simulink library "SUB_L4_Task_10ms_SUB_VELOCITYDISTCTRL"  (R2018a)
settings: Solver=VariableStepAuto  StartTime=0.0  StopTime=10.0  RelTol=1e-3
undefined symbols (not defined in the file or in its folder): DiscIntNeverNeededParam, ENUM_XBR_CONTROL_MODE_T, ENUM_XBR_EBI_MODE_T, ENUM_XBR_PASS_THROUGH_ACTIVE_T, ENUM_XBR_PRIORITY_T, magnitude
libraries: EmE_MBD_Blockset x14, simulink x6, PTC_MBDS_LIB x1
settings Model: Creator=Chris.Balton  LastModifiedBy=Chris.Balton

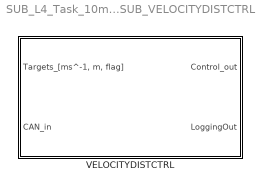
== system SUB_L4_Task_10ms_SUB_VELOCITYDISTCTRL ==
  VELOCITYDISTCTRL : Subsystem

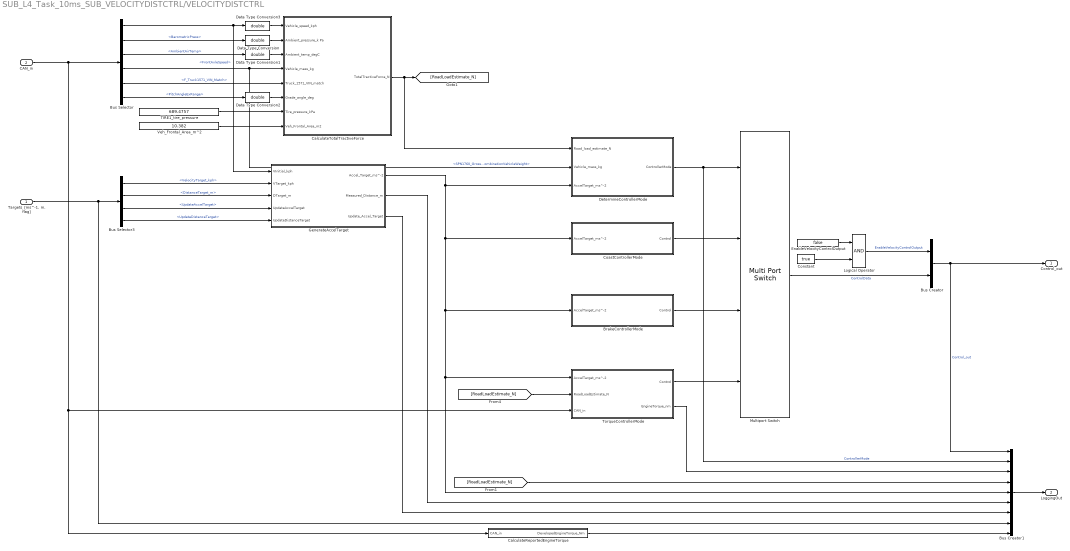
== system SUB_L4_Task_10ms_SUB_VELOCITYDISTCTRL/VELOCITYDISTCTRL ==
  "Targets_[ms^-1, m, flag]" : Inport
  CAN_in : Inport  Port=2
  BrakeControllerMode : Subsystem
  Bus Creator : BusCreator  Inputs=2
  Bus Creator1 : BusCreator  Inputs=9
  Bus Selector : BusSelector  OutputSignals=CAN.EBC2_0B.FrontAxleSpeed,CAN.AMB_00.BarometricPress,CAN.AMB_00.AmbientAirTemp,CAN.CVW_0B.SPN1760_GrossCombinationVehicleWeight,CAN.VI_00.F_Truck1571_VIN_Match,CAN.SSI2_03.PitchAngleExRange
  Bus Selector3 : BusSelector  OutputSignals=VelocityTarget_kph,DistanceTarget_m,UpdateAccelTarget,UpdateDistanceTarget
  CalculateReportedEngineTorque : Subsystem
  CalculateTotalTractiveForce : Subsystem
  CoastControllerMode : Subsystem
  Constant : Constant  Value=true  OutDataTypeStr=boolean
  Data Type Conversion{,1..3} (4 alike) : DataTypeConversion  OutDataTypeStr=double
      settings: AttributesFormatString=%<OutDataTypeStr>
  DetermineControllerMode : Subsystem
  EnableVelocityControlOutput : Constant  Value=false  OutDataTypeStr=boolean
  GenerateAccelTarget : Subsystem
  Logical Operator : Logic  OutDataTypeStr=boolean
  Multiport Switch : MultiPortSwitch
  TIRE1_tire_pressure : Constant  Value=689.4757
  TorqueControllerMode : Subsystem
  Veh_Frontal_Area_m^2 : Constant  Value=10.382
  Control_out : Outport
  LoggingOut : Outport  Port=2
  wires:
  Bus Selector3/4 -> GenerateAccelTarget/5(UpdateDistanceTarget)  "<UpdateDistanceTarget>"
  [RoadLoadEstimate_N] -> Bus Creator1/4
  CalculateReportedEngineTorque/1(DevelopedEngineTorque_Nm) -> Bus Creator1/9
  GenerateAccelTarget/2(Measured_Distance_m) -> Bus Creator1/6
  GenerateAccelTarget/3(Update_Accel_Target) -> Bus Creator1/7
  Constant/1 -> Logical Operator/2
  EnableVelocityControlOutput/1 -> Logical Operator/1
  Bus Creator1/1 -> LoggingOut/1
  TorqueControllerMode/2(EngineTorque_nm) -> Bus Creator1/3
  Logical Operator/1 -> Bus Creator/1  "EnableVelocityControlOutput"
  Bus Creator/1 -> Control_out/1, Bus Creator1/1  "Control_out"
  CAN_in/1 -> Bus Selector/1, CalculateReportedEngineTorque/1(CAN_in), TorqueControllerMode/3(CAN_in)
  Bus Selector/4 -> DetermineControllerMode/2(Vehicle_mass_kg), CalculateTotalTractiveForce/4(Vehicle_mass_kg)  "<SPN1760_GrossCombinationVehicleWeight>"
  Bus Selector/3 -> Data Type Conversion1/1  "<AmbientAirTemp>"
  Bus Selector3/3 -> GenerateAccelTarget/4(UpdateAccelTarget)  "<UpdateAccelTarget>"
  Data Type Conversion3/1 -> CalculateTotalTractiveForce/1(Vehicle_speed_kph)
  Bus Selector/1 -> Data Type Conversion3/1, GenerateAccelTarget/1(VInitial_kph)  "<FrontAxleSpeed>"
  Data Type Conversion1/1 -> CalculateTotalTractiveForce/3(Ambient_temp_degC)
  Data Type Conversion/1 -> CalculateTotalTractiveForce/2(Ambient_pressure_k Pa)
  Bus Selector3/2 -> GenerateAccelTarget/3(DTarget_m)  "<DistanceTarget_m>"
  Bus Selector3/1 -> GenerateAccelTarget/2(VTarget_kph)  "<VelocityTarget_kph>"
  Bus Selector/6 -> Data Type Conversion2/1  "<PitchAngleExRange>"
  TIRE1_tire_pressure/1 -> CalculateTotalTractiveForce/7(Tire_pressure_kPa)
  Veh_Frontal_Area_m^2/1 -> CalculateTotalTractiveForce/8(Veh_Frontal_Area_m2)
  "Targets_[ms^-1, m, flag]"/1 -> Bus Creator1/8, Bus Selector3/1
  Bus Selector/5 -> CalculateTotalTractiveForce/5(Truck_1571_VIN_match)  "<F_Truck1571_VIN_Match>"
  Bus Selector/2 -> Data Type Conversion/1  "<BarometricPress>"
  DetermineControllerMode/1(ControllerMode) -> Multiport Switch/1, Bus Creator1/2  "ControllerMode"
  GenerateAccelTarget/1(Accel_Target_ms^-2) -> Bus Creator1/5, TorqueControllerMode/1(AccelTarget_ms^-2), BrakeControllerMode/1(AccelTarget_ms^-2), CoastControllerMode/1(AccelTarget_ms^-2), DetermineControllerMode/3(AccelTarget_ms^-2)
  [RoadLoadEstimate_N] -> TorqueControllerMode/2(RoadLoadEstimate_N)
  CalculateTotalTractiveForce/1(TotalTractiveForce_N) -> DetermineControllerMode/1(Road_load_estimate_N), [RoadLoadEstimate_N]
  Multiport Switch/1 -> Bus Creator/2  "ControlData"
  TorqueControllerMode/1(Control) -> Multiport Switch/4
  BrakeControllerMode/1(Control) -> Multiport Switch/3
  CoastControllerMode/1(Control) -> Multiport Switch/2
  Data Type Conversion2/1 -> CalculateTotalTractiveForce/6(Grade_angle_deg)

== system SUB_L4_Task_10ms_SUB_VELOCITYDISTCTRL/VELOCITYDISTCTRL/BrakeControllerMode ==
  AccelTarget_ms^-2 : Inport
  Accel_pedal_coast : Constant  Value=0
  Bus Creator : BusCreator  Inputs=2
  Bus Creator1 : BusCreator  Inputs=7
  Gain : Gain
  XBRControlMode : Constant  Value=ENUM_XBR_CONTROL_MODE_T.ACCEL_CTRL_WITH_MAX_MODE
  XBREnduranceBrakeIntegrationMode : Constant  Value=ENUM_XBR_EBI_MODE_T.EBI_ALLOWED
  XBRPassThroughActiveOVR : Constant  Value=ENUM_XBR_PASS_THROUGH_ACTIVE_T.ACTIVE
  XBRPassThroughEnabled : Constant
  XBRPriority : Constant  Value=ENUM_XBR_PRIORITY_T.MEDIUM_PRIORITY
  XBRUrgency : Constant  Value=25
  Control : Outport
  wires:
  AccelTarget_ms^-2/1 -> Gain/1  "AccelTarget_ms^-2"
  Bus Creator1/1 -> Bus Creator/1  "XBR_data"
  Gain/1 -> Bus Creator1/1  "XBRExternalAccelDemand"
  XBRPassThroughActiveOVR/1 -> Bus Creator1/5  "XBRPassThroughActive"
  XBREnduranceBrakeIntegrationMode/1 -> Bus Creator1/2  "XBREnduranceBrakeIntegrationMode"
  XBRUrgency/1 -> Bus Creator1/6  "XBRUrgency"
  XBRControlMode/1 -> Bus Creator1/4  "XBRControlMode"
  XBRPriority/1 -> Bus Creator1/3  "XBRPriority"
  XBRPassThroughEnabled/1 -> Bus Creator1/7  "XBRPassThroughEnabled"
  Bus Creator/1 -> Control/1  "ControlData"
  Accel_pedal_coast/1 -> Bus Creator/2  "AcceleratorPedalPosOut"

== system SUB_L4_Task_10ms_SUB_VELOCITYDISTCTRL/VELOCITYDISTCTRL/CalculateReportedEngineTorque ==
  CAN_in : Inport
  Add : Sum  OutDataTypeStr=double  InputSameDT=on
  Bus Selector : BusSelector  OutputSignals=CAN.EC1_00.SPN544_EngineReferenceTorque,CAN.EEC1_00.ActlEngPrcntTrqueHighResolution,CAN.EEC1_00.ActualEngPercentTorque
  ConvToPercent : Constant  Value=0.01
  Data Type Conversion : DataTypeConversion  OutDataTypeStr=double
  Product : Product  Inputs=3  InputSameDT=on
  DevelopedEngineTorque_Nm : Outport
      settings: AttributesFormatString=IC: %<InitialOutput>\nDisabled value: %<OutputWhenDisabled>
  wires:
  ConvToPercent/1 -> Product/3
  Product/1 -> DevelopedEngineTorque_Nm/1  "DevelopedEngineTorque_Nm"
  Add/1 -> Product/2  "EnginePercentTorque"
  Bus Selector/3 -> Add/2  "<ActualEngPercentTorque>"
  Bus Selector/2 -> Add/1  "<ActlEngPrcntTrqueHighResolution>"
  Bus Selector/1 -> Data Type Conversion/1  "<SPN544_EngineReferenceTorque>"
  CAN_in/1 -> Bus Selector/1
  Data Type Conversion/1 -> Product/1

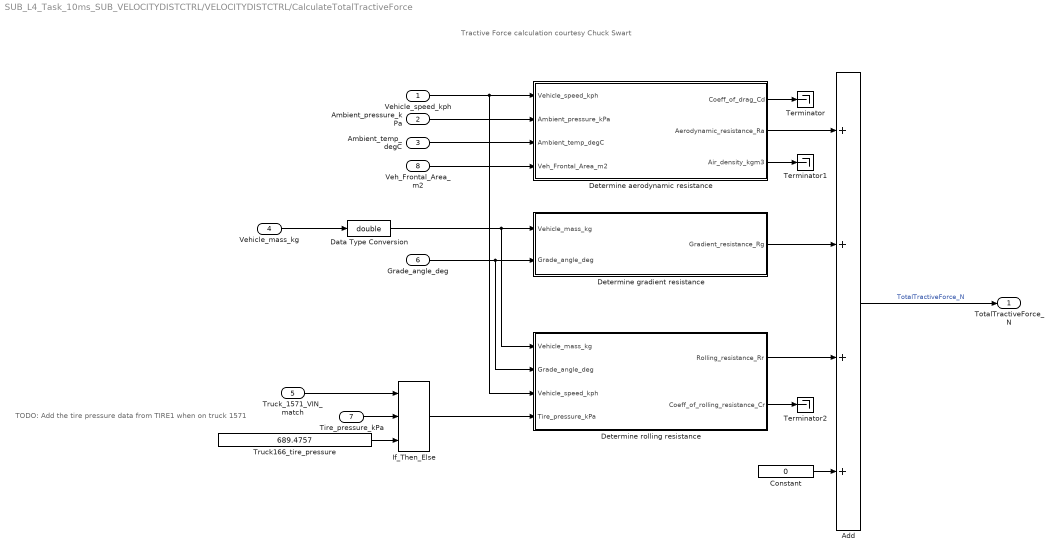
== system SUB_L4_Task_10ms_SUB_VELOCITYDISTCTRL/VELOCITYDISTCTRL/CalculateTotalTractiveForce ==
  note: TODO: Add the tire pressure data from TIRE1 when on truck 1571
  note: Tractive Force calculation courtesy Chuck Swart
  Vehicle_speed_kph : Inport
  Ambient_pressure_k Pa : Inport  Port=2
  Ambient_temp_degC : Inport  Port=3
  Vehicle_mass_kg : Inport  Port=4
  Truck_1571_VIN_match : Inport  Port=5
  Grade_angle_deg : Inport  Port=6
  Tire_pressure_kPa : Inport  Port=7
  Veh_Frontal_Area_m2 : Inport  Port=8
  Add : Sum  Inputs=++++  InputSameDT=on
  Constant : Constant  Value=0
  Data Type Conversion : DataTypeConversion  OutDataTypeStr=double
  Determine aerodynamic resistance : Subsystem
  Determine gradient resistance : Subsystem
  Determine rolling resistance : Subsystem
  If_Then_Else : EmE_MBD_Blockset/Signal Routing/If_Then_Else
      settings: SourceProductName=PACCAR EmE MBD Blockset
  Terminator : Terminator
  Terminator1 : Terminator
  Terminator2 : Terminator
  Truck166_tire_pressure : Constant  Value=689.4757
  TotalTractiveForce_N : Outport
  wires:
  If_Then_Else/1 -> Determine rolling resistance/4(Tire_pressure_kPa)
  Determine rolling resistance/2(Coeff_of_rolling_resistance_Cr) -> Terminator2/1
  Determine rolling resistance/1(Rolling_resistance_Rr) -> Add/3
  Ambient_pressure_k Pa/1 -> Determine aerodynamic resistance/2(Ambient_pressure_kPa)
  Add/1 -> TotalTractiveForce_N/1  "TotalTractiveForce_N"
  Vehicle_speed_kph/1 -> Determine rolling resistance/3(Vehicle_speed_kph), Determine aerodynamic resistance/1(Vehicle_speed_kph)
  Ambient_temp_degC/1 -> Determine aerodynamic resistance/3(Ambient_temp_degC)
  Determine aerodynamic resistance/1(Coeff_of_drag_Cd) -> Terminator/1
  Veh_Frontal_Area_m2/1 -> Determine aerodynamic resistance/4(Veh_Frontal_Area_m2)
  Constant/1 -> Add/4
  Vehicle_mass_kg/1 -> Data Type Conversion/1
  Grade_angle_deg/1 -> Determine rolling resistance/2(Grade_angle_deg), Determine gradient resistance/2(Grade_angle_deg)
  Determine gradient resistance/1(Gradient_resistance_Rg) -> Add/2
  Determine aerodynamic resistance/3(Air_density_kgm3) -> Terminator1/1
  Determine aerodynamic resistance/2(Aerodynamic_resistance_Ra) -> Add/1
  Tire_pressure_kPa/1 -> If_Then_Else/2
  Truck166_tire_pressure/1 -> If_Then_Else/3
  Truck_1571_VIN_match/1 -> If_Then_Else/1
  Data Type Conversion/1 -> Determine rolling resistance/1(Vehicle_mass_kg), Determine gradient resistance/1(Vehicle_mass_kg)

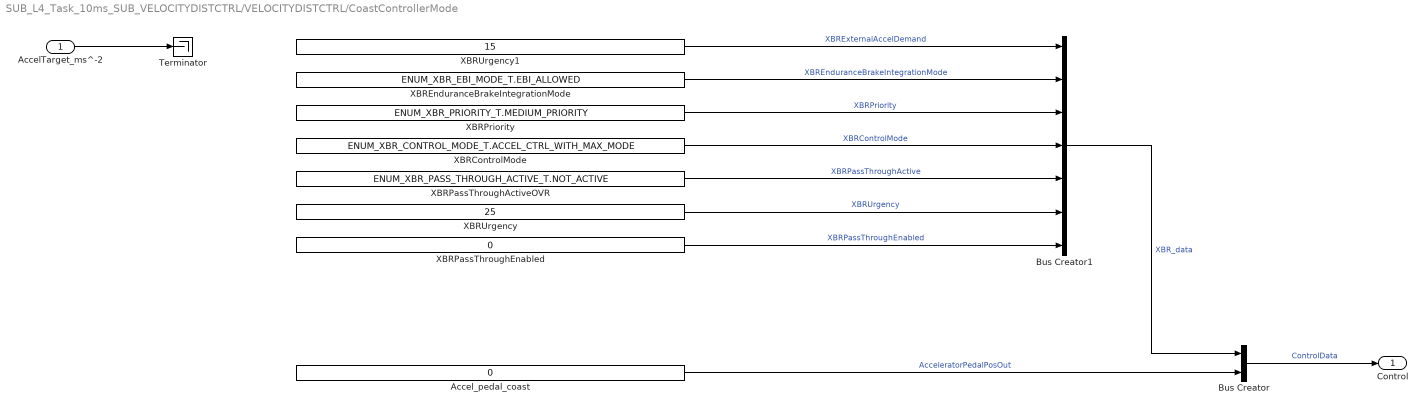
== system SUB_L4_Task_10ms_SUB_VELOCITYDISTCTRL/VELOCITYDISTCTRL/CoastControllerMode ==
  AccelTarget_ms^-2 : Inport
  Accel_pedal_coast : Constant  Value=0
  Bus Creator : BusCreator  Inputs=2
  Bus Creator1 : BusCreator  Inputs=7
  Terminator : Terminator
  XBRControlMode : Constant  Value=ENUM_XBR_CONTROL_MODE_T.ACCEL_CTRL_WITH_MAX_MODE
  XBREnduranceBrakeIntegrationMode : Constant  Value=ENUM_XBR_EBI_MODE_T.EBI_ALLOWED
  XBRPassThroughActiveOVR : Constant  Value=ENUM_XBR_PASS_THROUGH_ACTIVE_T.NOT_ACTIVE
  XBRPassThroughEnabled : Constant  Value=0
  XBRPriority : Constant  Value=ENUM_XBR_PRIORITY_T.MEDIUM_PRIORITY
  XBRUrgency : Constant  Value=25
  XBRUrgency1 : Constant  Value=15
  Control : Outport
  wires:
  Bus Creator1/1 -> Bus Creator/1  "XBR_data"
  XBRUrgency1/1 -> Bus Creator1/1  "XBRExternalAccelDemand"
  XBRPassThroughActiveOVR/1 -> Bus Creator1/5  "XBRPassThroughActive"
  XBREnduranceBrakeIntegrationMode/1 -> Bus Creator1/2  "XBREnduranceBrakeIntegrationMode"
  XBRUrgency/1 -> Bus Creator1/6  "XBRUrgency"
  XBRControlMode/1 -> Bus Creator1/4  "XBRControlMode"
  XBRPriority/1 -> Bus Creator1/3  "XBRPriority"
  XBRPassThroughEnabled/1 -> Bus Creator1/7  "XBRPassThroughEnabled"
  AccelTarget_ms^-2/1 -> Terminator/1
  Bus Creator/1 -> Control/1  "ControlData"
  Accel_pedal_coast/1 -> Bus Creator/2  "AcceleratorPedalPosOut"

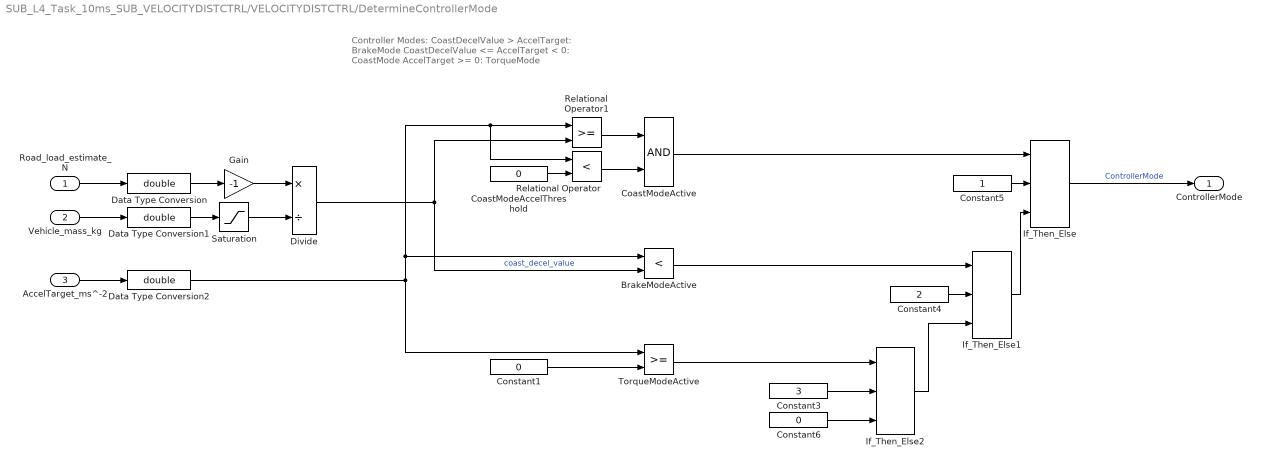
== system SUB_L4_Task_10ms_SUB_VELOCITYDISTCTRL/VELOCITYDISTCTRL/DetermineControllerMode ==
  note: Controller Modes:
      |
      | CoastDecelValue  >  AccelTarget:         BrakeMode
      | CoastDecelValue <= AccelTarget < 0:   CoastMode
      |                                  AccelTarget >= 0: TorqueMode
  Road_load_estimate_N : Inport
  Vehicle_mass_kg : Inport  Port=2
  AccelTarget_ms^-2 : Inport  Port=3
  BrakeModeActive : RelationalOperator  Operator=<  OutDataTypeStr=boolean  RndMeth=Nearest
  CoastModeAccelThreshold : Constant  Value=0
  CoastModeActive : Logic  AllPortsSameDT=off  OutDataTypeStr=boolean
  Constant1 : Constant  Value=0  SampleTime=-1
  Constant3 : Constant  Value=3  SampleTime=0.01
  Constant4 : Constant  Value=2  SampleTime=0.01
  Constant5 : Constant  SampleTime=0.01
  Constant6 : Constant  Value=0  SampleTime=0.01
  Data Type Conversion : DataTypeConversion  OutDataTypeStr=double
  Data Type Conversion1 : DataTypeConversion  OutDataTypeStr=double
  Data Type Conversion2 : DataTypeConversion  OutDataTypeStr=double
  Divide : Product  Inputs=*/  InputSameDT=on
  Gain : Gain  Gain=-1
  If_Then_Else : EmE_MBD_Blockset/Signal Routing/If_Then_Else
      settings: SourceProductName=PACCAR EmE MBD Blockset
  If_Then_Else1 : EmE_MBD_Blockset/Signal Routing/If_Then_Else
      settings: SourceProductName=PACCAR EmE MBD Blockset
  If_Then_Else2 : EmE_MBD_Blockset/Signal Routing/If_Then_Else
      settings: SourceProductName=PACCAR EmE MBD Blockset
  Relational Operator : RelationalOperator  Operator=<  OutDataTypeStr=boolean  RndMeth=Nearest
  Relational Operator1 : RelationalOperator  OutDataTypeStr=boolean  RndMeth=Nearest
  Saturation : Saturate  UpperLimit=50000  LowerLimit=1
  TorqueModeActive : RelationalOperator  OutDataTypeStr=boolean  RndMeth=Nearest
  ControllerMode : Outport
  wires:
  Road_load_estimate_N/1 -> Data Type Conversion/1
  Vehicle_mass_kg/1 -> Data Type Conversion1/1
  Saturation/1 -> Divide/2
  Gain/1 -> Divide/1
  Divide/1 -> BrakeModeActive/2, Relational Operator1/2  "coast_decel_value"
  If_Then_Else/1 -> ControllerMode/1  "ControllerMode"
  Constant6/1 -> If_Then_Else2/3
  Constant5/1 -> If_Then_Else/2
  Constant4/1 -> If_Then_Else1/2
  Constant3/1 -> If_Then_Else2/2
  If_Then_Else2/1 -> If_Then_Else1/3
  If_Then_Else1/1 -> If_Then_Else/3
  CoastModeAccelThreshold/1 -> Relational Operator/2
  Relational Operator1/1 -> CoastModeActive/1
  Relational Operator/1 -> CoastModeActive/2
  TorqueModeActive/1 -> If_Then_Else2/1
  BrakeModeActive/1 -> If_Then_Else1/1
  Constant1/1 -> TorqueModeActive/2
  AccelTarget_ms^-2/1 -> Data Type Conversion2/1
  CoastModeActive/1 -> If_Then_Else/1
  Data Type Conversion/1 -> Gain/1
  Data Type Conversion1/1 -> Saturation/1
  Data Type Conversion2/1 -> TorqueModeActive/1, BrakeModeActive/1, Relational Operator1/1, Relational Operator/1

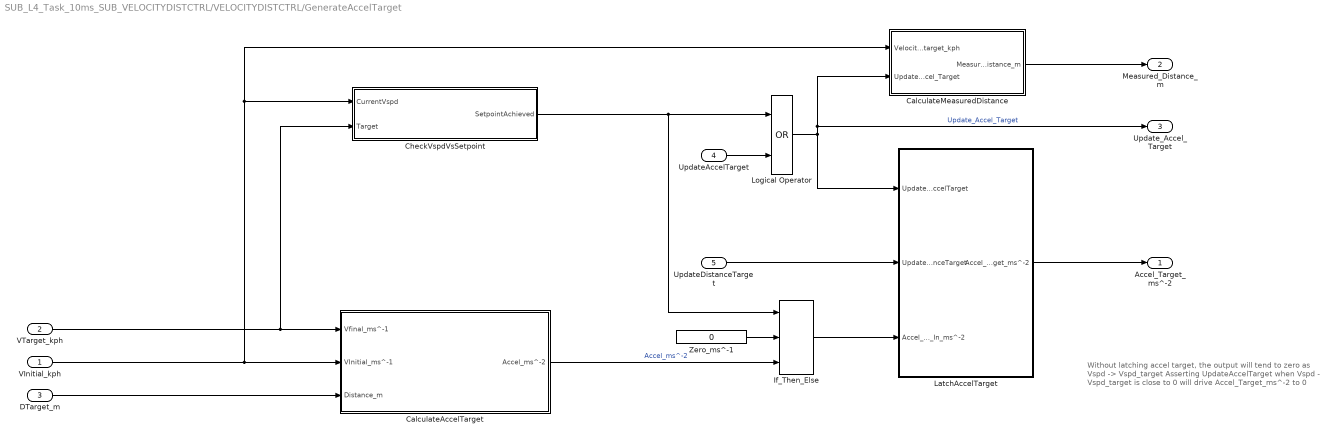
== system SUB_L4_Task_10ms_SUB_VELOCITYDISTCTRL/VELOCITYDISTCTRL/GenerateAccelTarget ==
  note: Without latching accel target, the output will tend to zero as Vspd -> Vspd_target
      |
      | Asserting UpdateAccelTarget when Vspd - Vspd_target is close to 0 will drive Accel_Target_ms^-2 to 0
  VInitial_kph : Inport
  VTarget_kph : Inport  Port=2
  DTarget_m : Inport  Port=3
  UpdateAccelTarget : Inport  Port=4
  UpdateDistanceTarget : Inport  Port=5
  CalculateAccelTarget : Subsystem
  CalculateMeasuredDistance : Subsystem
  CheckVspdVsSetpoint : Subsystem
  If_Then_Else : EmE_MBD_Blockset/Signal Routing/If_Then_Else
      settings: SourceProductName=PACCAR EmE MBD Blockset
  LatchAccelTarget : Subsystem
  Logical Operator : Logic  Operator=OR  OutDataTypeStr=boolean
  Zero_ms^-1 : Constant  Value=0
  Accel_Target_ms^-2 : Outport
  Measured_Distance_m : Outport  Port=2
  Update_Accel_Target : Outport  Port=3
  wires:
  UpdateDistanceTarget/1 -> LatchAccelTarget/2(UpdateDistanceTarget)
  CalculateMeasuredDistance/1(Measured_Distance_m) -> Measured_Distance_m/1
  CalculateAccelTarget/1(Accel_ms^-2) -> If_Then_Else/3  "Accel_ms^-2"
  DTarget_m/1 -> CalculateAccelTarget/3(Distance_m)
  If_Then_Else/1 -> LatchAccelTarget/3(Accel_Target_In_ms^-2)
  Zero_ms^-1/1 -> If_Then_Else/2
  UpdateAccelTarget/1 -> Logical Operator/2
  CheckVspdVsSetpoint/1(SetpointAchieved) -> Logical Operator/1, If_Then_Else/1
  LatchAccelTarget/1(Accel_Target_ms^-2) -> Accel_Target_ms^-2/1
  Logical Operator/1 -> LatchAccelTarget/1(UpdateAccelTarget), CalculateMeasuredDistance/2(Update_Accel_Target), Update_Accel_Target/1  "Update_Accel_Target"
  VInitial_kph/1 -> CalculateAccelTarget/2(VInitial_ms^-1), CheckVspdVsSetpoint/1(CurrentVspd), CalculateMeasuredDistance/1(Velocity_target_kph)
  VTarget_kph/1 -> CalculateAccelTarget/1(Vfinal_ms^-1), CheckVspdVsSetpoint/2(Target)

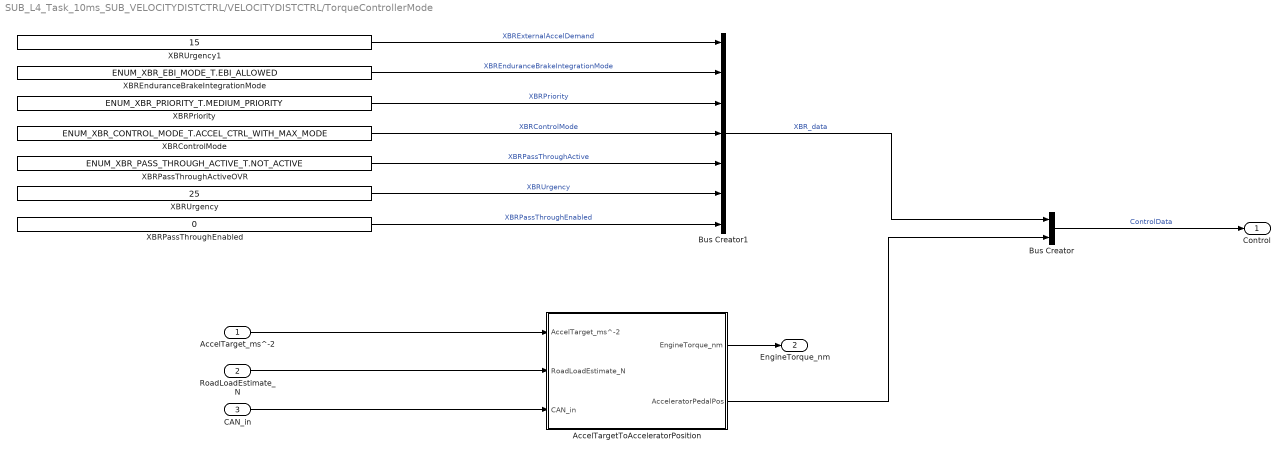
== system SUB_L4_Task_10ms_SUB_VELOCITYDISTCTRL/VELOCITYDISTCTRL/TorqueControllerMode ==
  AccelTarget_ms^-2 : Inport
  RoadLoadEstimate_N : Inport  Port=2
  CAN_in : Inport  Port=3
  AccelTargetToAcceleratorPosition : Subsystem
  Bus Creator : BusCreator  Inputs=2
  Bus Creator1 : BusCreator  Inputs=7
  XBRControlMode : Constant  Value=ENUM_XBR_CONTROL_MODE_T.ACCEL_CTRL_WITH_MAX_MODE
  XBREnduranceBrakeIntegrationMode : Constant  Value=ENUM_XBR_EBI_MODE_T.EBI_ALLOWED
  XBRPassThroughActiveOVR : Constant  Value=ENUM_XBR_PASS_THROUGH_ACTIVE_T.NOT_ACTIVE
  XBRPassThroughEnabled : Constant  Value=0
  XBRPriority : Constant  Value=ENUM_XBR_PRIORITY_T.MEDIUM_PRIORITY
  XBRUrgency : Constant  Value=25
  XBRUrgency1 : Constant  Value=15
  Control : Outport
  EngineTorque_nm : Outport  Port=2
  wires:
  AccelTargetToAcceleratorPosition/1(EngineTorque_nm) -> EngineTorque_nm/1
  CAN_in/1 -> AccelTargetToAcceleratorPosition/3(CAN_in)
  RoadLoadEstimate_N/1 -> AccelTargetToAcceleratorPosition/2("RoadLoadEstimate_N ")
  AccelTarget_ms^-2/1 -> AccelTargetToAcceleratorPosition/1(AccelTarget_ms^-2)
  Bus Creator1/1 -> Bus Creator/1  "XBR_data"
  XBRUrgency1/1 -> Bus Creator1/1  "XBRExternalAccelDemand"
  XBRPassThroughActiveOVR/1 -> Bus Creator1/5  "XBRPassThroughActive"
  XBREnduranceBrakeIntegrationMode/1 -> Bus Creator1/2  "XBREnduranceBrakeIntegrationMode"
  XBRUrgency/1 -> Bus Creator1/6  "XBRUrgency"
  XBRControlMode/1 -> Bus Creator1/4  "XBRControlMode"
  XBRPriority/1 -> Bus Creator1/3  "XBRPriority"
  XBRPassThroughEnabled/1 -> Bus Creator1/7  "XBRPassThroughEnabled"
  Bus Creator/1 -> Control/1  "ControlData"
  AccelTargetToAcceleratorPosition/2(AcceleratorPedalPos) -> Bus Creator/2

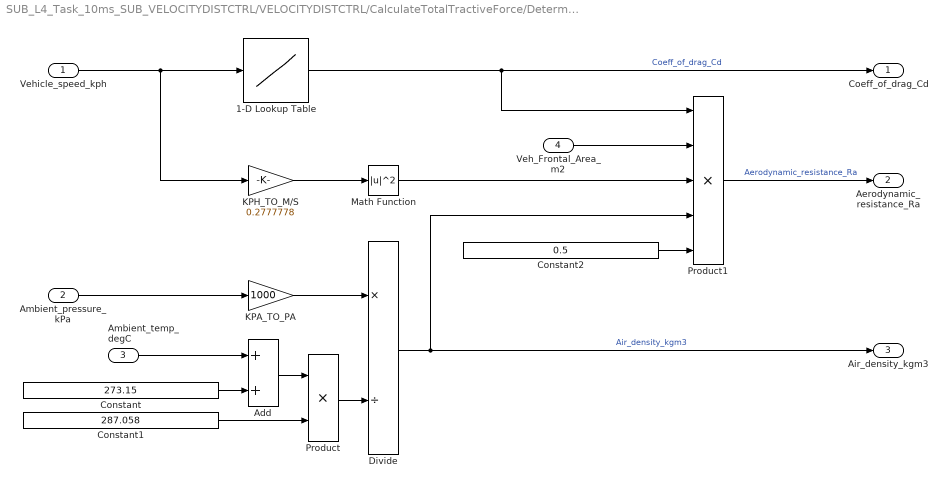
== system SUB_L4_Task_10ms_SUB_VELOCITYDISTCTRL/VELOCITYDISTCTRL/CalculateTotalTractiveForce/Determine aerodynamic resistance ==
  Vehicle_speed_kph : Inport
  Ambient_pressure_kPa : Inport  Port=2
  Ambient_temp_degC : Inport  Port=3
  Veh_Frontal_Area_m2 : Inport  Port=4
  1-D Lookup Table : Lookup_n-D  NumberOfTableDimensions=1  BreakpointsForDimension1=[0 1 200]  Table=[0 0.5779 0.5779]  TableDataTypeStr=Inherit: Inherit from 'Table data'  ExtrapMethod=Clip  UseLastTableValue=on  OutDataTypeStr=Inherit: Inherit from 'Table data'  InputSameDT=on
      settings: AttributesFormatString=|
      | X: %<BreakpointsForDimension1>
      | Y: %<Table>
  Add : Sum  InputSameDT=on
  Constant : Constant  Value=273.15
  Constant1 : Constant  Value=287.058
  Constant2 : Constant  Value=0.5
  Divide : Product  Inputs=*/  InputSameDT=on
  KPA_TO_PA : Gain  Gain=1000  OutDataTypeStr=double
  KPH_TO_M/S : Gain  Gain=0.2777778  OutDataTypeStr=double
  Math Function : Math  Operator=magnitude^2  SaturateOnIntegerOverflow=on
  Product : Product  InputSameDT=on
  Product1 : Product  Inputs=5  InputSameDT=on
  Coeff_of_drag_Cd : Outport
  Aerodynamic_resistance_Ra : Outport  Port=2
  Air_density_kgm3 : Outport  Port=3
  wires:
  KPA_TO_PA/1 -> Divide/1
  Ambient_temp_degC/1 -> Add/1
  Constant/1 -> Add/2
  Add/1 -> Product/1
  Constant1/1 -> Product/2
  Product/1 -> Divide/2
  Constant2/1 -> Product1/5
  Divide/1 -> Product1/4, Air_density_kgm3/1  "Air_density_kgm3"
  Veh_Frontal_Area_m2/1 -> Product1/2
  Math Function/1 -> Product1/3
  1-D Lookup Table/1 -> Coeff_of_drag_Cd/1, Product1/1  "Coeff_of_drag_Cd"
  Product1/1 -> Aerodynamic_resistance_Ra/1  "Aerodynamic_resistance_Ra"
  Vehicle_speed_kph/1 -> KPH_TO_M/S/1, 1-D Lookup Table/1
  Ambient_pressure_kPa/1 -> KPA_TO_PA/1
  KPH_TO_M/S/1 -> Math Function/1

== system SUB_L4_Task_10ms_SUB_VELOCITYDISTCTRL/VELOCITYDISTCTRL/CalculateTotalTractiveForce/Determine gradient resistance ==
  Vehicle_mass_kg : Inport
  Grade_angle_deg : Inport  Port=2
  Constant1 : Constant  Value=9.807
  Constant2 : Constant  Value=pi
  Constant3 : Constant  Value=180
  Data Type Conversion Inherited : simulink/Signal Attributes/Data Type Conversion Inherited  ConvertRealWorld=Real World Value  DoSatur=off
      settings: SourceProductName=Simulink  SourceProductBaseCode=SL
  Data Type Conversion Inherited1 : simulink/Signal Attributes/Data Type Conversion Inherited  ConvertRealWorld=Real World Value  DoSatur=off
      settings: SourceProductName=Simulink  SourceProductBaseCode=SL
  Data Type Conversion Inherited2 : simulink/Signal Attributes/Data Type Conversion Inherited  ConvertRealWorld=Real World Value  DoSatur=off
      settings: SourceProductName=Simulink  SourceProductBaseCode=SL
  Divide : Product  Inputs=**/  InputSameDT=on
  Product1 : Product  Inputs=3  InputSameDT=on
  Trigonometric Function : Trigonometry
  Gradient_resistance_Rg : Outport
  wires:
  Constant1/1 -> Data Type Conversion Inherited2/2
  Trigonometric Function/1 -> Product1/2
  Constant2/1 -> Data Type Conversion Inherited/2
  Divide/1 -> Trigonometric Function/1  "grade_angle_radians"
  Product1/1 -> Gradient_resistance_Rg/1  "Gradient_resistance_Rg"
  Vehicle_mass_kg/1 -> Data Type Conversion Inherited2/1, Product1/1
  Grade_angle_deg/1 -> Data Type Conversion Inherited1/1, Data Type Conversion Inherited/1, Divide/1
  Data Type Conversion Inherited/1 -> Divide/2
  Data Type Conversion Inherited1/1 -> Divide/3
  Constant3/1 -> Data Type Conversion Inherited1/2
  Data Type Conversion Inherited2/1 -> Product1/3

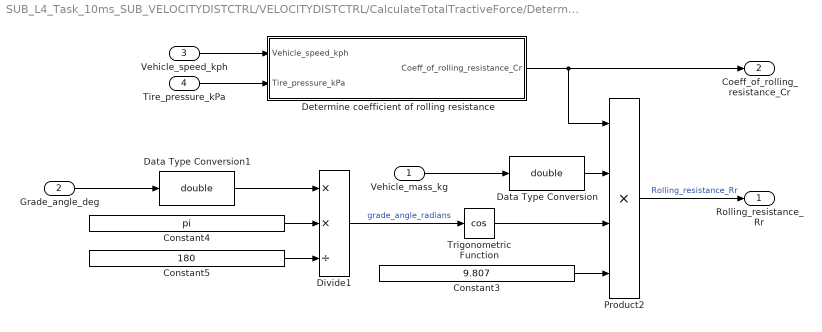
== system SUB_L4_Task_10ms_SUB_VELOCITYDISTCTRL/VELOCITYDISTCTRL/CalculateTotalTractiveForce/Determine rolling resistance ==
  Vehicle_mass_kg : Inport
  Grade_angle_deg : Inport  Port=2
  Vehicle_speed_kph : Inport  Port=3
  Tire_pressure_kPa : Inport  Port=4
  Constant3 : Constant  Value=9.807
  Constant4 : Constant  Value=pi
  Constant5 : Constant  Value=180
  Data Type Conversion : DataTypeConversion  OutDataTypeStr=double
  Data Type Conversion1 : DataTypeConversion  OutDataTypeStr=double
  Determine coefficient of rolling resistance : Subsystem
  Divide1 : Product  Inputs=**/  InputSameDT=on
  Product2 : Product  Inputs=4  InputSameDT=on
  Trigonometric Function : Trigonometry  Operator=cos
  Rolling_resistance_Rr : Outport
  Coeff_of_rolling_resistance_Cr : Outport  Port=2
  wires:
  Constant3/1 -> Product2/4
  Trigonometric Function/1 -> Product2/3
  Constant5/1 -> Divide1/3
  Constant4/1 -> Divide1/2
  Divide1/1 -> Trigonometric Function/1  "grade_angle_radians"
  Vehicle_mass_kg/1 -> Data Type Conversion/1
  Grade_angle_deg/1 -> Data Type Conversion1/1
  Product2/1 -> Rolling_resistance_Rr/1  "Rolling_resistance_Rr"
  Vehicle_speed_kph/1 -> Determine coefficient of rolling resistance/1(Vehicle_speed_kph)
  Tire_pressure_kPa/1 -> Determine coefficient of rolling resistance/2(Tire_pressure_kPa)
  Determine coefficient of rolling resistance/1(Coeff_of_rolling_resistance_Cr) -> Coeff_of_rolling_resistance_Cr/1, Product2/1
  Data Type Conversion/1 -> Product2/2
  Data Type Conversion1/1 -> Divide1/1

== system SUB_L4_Task_10ms_SUB_VELOCITYDISTCTRL/VELOCITYDISTCTRL/GenerateAccelTarget/CalculateAccelTarget ==
  note: For very small D, the accel target will be huge. Saturating this against a minimum value > 0 will ensure bounded outputs when distance feedback is introduced.
  Vfinal_ms^-1 : Inport
  VInitial_ms^-1 : Inport  Port=2
  Distance_m : Inport  Port=3
  Data Type Conversion2 : DataTypeConversion  OutDataTypeStr=double
      settings: AttributesFormatString=%<OutDataTypeStr>
  Divide : Product  Inputs=*/  OutDataTypeStr=double
  Gain : Gain  Gain=2
  Math Function : Math  Operator=square  SaturateOnIntegerOverflow=on
  Math Function1 : Math  Operator=square  SaturateOnIntegerOverflow=on
  Saturation : Saturate  UpperLimit=inf  LowerLimit=5
  Sum : Sum  Inputs=+-
  kph_to_m/s : Gain  Gain=0.277778
  kph_to_m/s1 : Gain  Gain=0.277778
  Accel_ms^-2 : Outport
  wires:
  Vfinal_ms^-1/1 -> kph_to_m/s1/1  "Vfinal_ms^-1"
  VInitial_ms^-1/1 -> Data Type Conversion2/1  "VInitial_ms^-1"
  Math Function/1 -> Sum/1
  Math Function1/1 -> Sum/2
  Sum/1 -> Divide/1
  Gain/1 -> Divide/2
  Saturation/1 -> Gain/1
  kph_to_m/s/1 -> Math Function1/1
  Distance_m/1 -> Saturation/1
  kph_to_m/s1/1 -> Math Function/1
  Data Type Conversion2/1 -> kph_to_m/s/1
  Divide/1 -> Accel_ms^-2/1  "Accel_ms^-2"

== system SUB_L4_Task_10ms_SUB_VELOCITYDISTCTRL/VELOCITYDISTCTRL/GenerateAccelTarget/CalculateMeasuredDistance ==
  Velocity_target_kph : Inport
  Update_Accel_Target : Inport  Port=2
  Discrete-Time Integrator : DiscreteIntegrator  ExternalReset=rising  SampleTime=-1  ICPrevOutput=DiscIntNeverNeededParam  ICPrevScaledInput=DiscIntNeverNeededParam
  Gain : Gain  Gain=0.27778
  Measured_Distance_m : Outport
  wires:
  Velocity_target_kph/1 -> Gain/1
  Update_Accel_Target/1 -> Discrete-Time Integrator/2
  Discrete-Time Integrator/1 -> Measured_Distance_m/1  "Measured_Distance_m"
  Gain/1 -> Discrete-Time Integrator/1  "velocity_ms^-1"

== system SUB_L4_Task_10ms_SUB_VELOCITYDISTCTRL/VELOCITYDISTCTRL/GenerateAccelTarget/CheckVspdVsSetpoint ==
  CurrentVspd : Inport
  Target : Inport  Port=2
  Abs : Abs
  Compare To Constant : simulink/Logic and Bit Operations/Compare To Constant  relop=<=  const=0.1  OutDataTypeStr=boolean
  Rising_edge : EmE_MBD_Blockset/Discontinuities/Rising_edge  initact=off
      settings: AttributesFormatString=Action on IC: %<initact>  SourceProductName=PACCAR EmE MBD Blockset
  Subtract : Sum  Inputs=+-
  SetpointAchieved : Outport
  wires:
  Rising_edge/1 -> SetpointAchieved/1
  Compare To Constant/1 -> Rising_edge/1
  Subtract/1 -> Abs/1
  Target/1 -> Subtract/1
  Abs/1 -> Compare To Constant/1
  CurrentVspd/1 -> Subtract/2

== system SUB_L4_Task_10ms_SUB_VELOCITYDISTCTRL/VELOCITYDISTCTRL/GenerateAccelTarget/LatchAccelTarget ==
  UpdateAccelTarget : Inport
  UpdateDistanceTarget : Inport  Port=2
  Accel_Target_In_ms^-2 : Inport  Port=3
  If_Then_Else : EmE_MBD_Blockset/Signal Routing/If_Then_Else
      settings: SourceProductName=PACCAR EmE MBD Blockset
  Logical Operator : Logic  Operator=OR  OutDataTypeStr=boolean
  Unit_Delay : UnitDelay  SampleTime=-1
      settings: AttributesFormatString=IC: %<vinit>
  Accel_Target_ms^-2 : Outport
  wires:
  Logical Operator/1 -> If_Then_Else/1
  UpdateDistanceTarget/1 -> Logical Operator/1
  Accel_Target_In_ms^-2/1 -> If_Then_Else/2
  UpdateAccelTarget/1 -> Logical Operator/2
  If_Then_Else/1 -> Accel_Target_ms^-2/1, Unit_Delay/1  "Accel_Target_ms^-2"
  Unit_Delay/1 -> If_Then_Else/3

== system SUB_L4_Task_10ms_SUB_VELOCITYDISTCTRL/VELOCITYDISTCTRL/TorqueControllerMode/AccelTargetToAcceleratorPosition ==
  AccelTarget_ms^-2 : Inport
  "RoadLoadEstimate_N " : Inport  Port=2
  CAN_in : Inport  Port=3
  AccelTargetToEngineTorque : Subsystem
  EngineTorqueToAccelPedalPos : Subsystem
  EngineTorque_nm : Outport
  AcceleratorPedalPos : Outport  Port=2
  wires:
  CAN_in/1 -> EngineTorqueToAccelPedalPos/2(Espd_rpm), AccelTargetToEngineTorque/3(CAN_In)
  "RoadLoadEstimate_N "/1 -> AccelTargetToEngineTorque/2("RoadLoadEstimate_N ")
  EngineTorqueToAccelPedalPos/1(AcceleratorPedalPosOut) -> AcceleratorPedalPos/1
  AccelTargetToEngineTorque/1(EngineTorque_Nm) -> EngineTorqueToAccelPedalPos/1(EngineTorque_Nm), EngineTorque_nm/1
  AccelTarget_ms^-2/1 -> AccelTargetToEngineTorque/1(AccelTarget_ms^-2)

== system SUB_L4_Task_10ms_SUB_VELOCITYDISTCTRL/VELOCITYDISTCTRL/CalculateTotalTractiveForce/Determine rolling resistance/Determine coefficient of rolling resistance ==
  Vehicle_speed_kph : Inport
  Tire_pressure_kPa : Inport  Port=2
  Add : Sum  InputSameDT=on
  Add1 : Sum  InputSameDT=on
  Constant : Constant  Value=0.005
  Constant1 : Constant  Value=0.01
  Constant2 : Constant  Value=0.0095
  Constant6 : Constant  Value=100
  Divide : Product  Inputs=*/  InputSameDT=on
  Divide2 : Product  Inputs=**/  InputSameDT=on
  KPA_TO_BAR : Gain  Gain=0.01
  Math Function : Math  Operator=magnitude^2  SaturateOnIntegerOverflow=on
  Coeff_of_rolling_resistance_Cr : Outport
  wires:
  Constant1/1 -> Add/1
  Constant6/1 -> Divide2/3
  Constant2/1 -> Divide2/1
  Constant/1 -> Add1/1
  Add/1 -> Divide/1
  Add1/1 -> Coeff_of_rolling_resistance_Cr/1  "Coeff_of_rolling_resistance_Cr"
  Math Function/1 -> Add/2
  Divide2/1 -> Math Function/1
  KPA_TO_BAR/1 -> Divide/2
  Divide/1 -> Add1/2
  Tire_pressure_kPa/1 -> KPA_TO_BAR/1
  Vehicle_speed_kph/1 -> Divide2/2

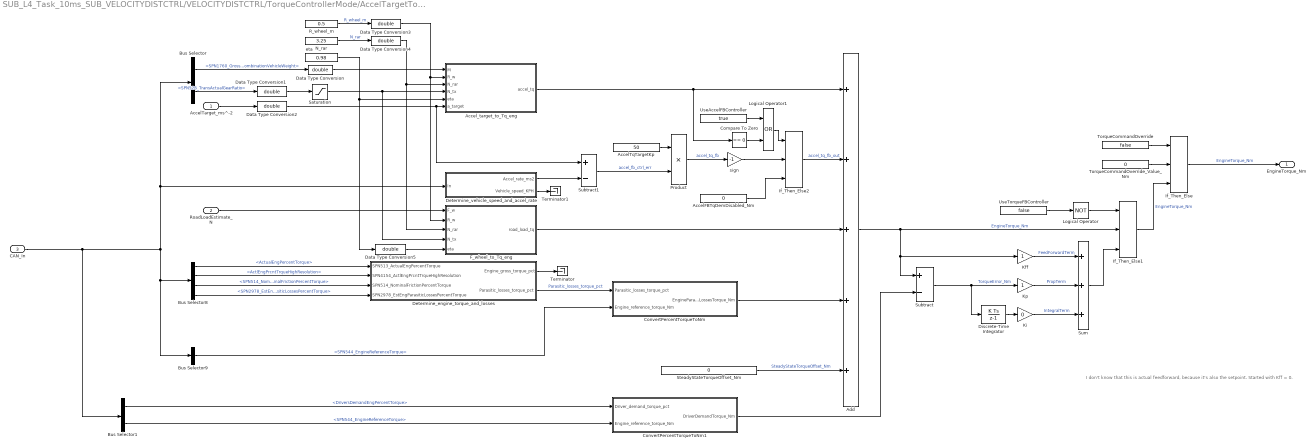
== system SUB_L4_Task_10ms_SUB_VELOCITYDISTCTRL/VELOCITYDISTCTRL/TorqueControllerMode/AccelTargetToAcceleratorPosition/AccelTargetToEngineTorque ==
  note: I don't know that this is actual feedforward, because it's also the setpoint. Started with Kff = 0.
  AccelTarget_ms^-2 : Inport
  "RoadLoadEstimate_N " : Inport  Port=2
  CAN_In : Inport  Port=3
  AccelFBTqDemDisabled_Nm : Constant  Value=0
  AccelTqTargetKp : Constant  Value=50
  Accel_target_to_Tq_eng : MATLAB Function  TreatAsAtomicUnit=on
  Add : Sum  Inputs=+++++  AccumDataTypeStr=double  InputSameDT=on
  Bus Selector : BusSelector  OutputSignals=CAN.CVW_0B.SPN1760_GrossCombinationVehicleWeight,CAN.ETC2_03.SPN526_TransActualGearRatio
  Bus Selector1 : BusSelector  OutputSignals=CAN.EEC1_00.DriversDemandEngPercentTorque,CAN.EC1_00.SPN544_EngineReferenceTorque
  Bus Selector8 : BusSelector  OutputSignals=CAN.EEC1_00.ActualEngPercentTorque,CAN.EEC1_00.ActlEngPrcntTrqueHighResolution,CAN.EEC3_00.SPN514_NominalFrictionPercentTorque,CAN.EEC3_00.SPN2978_EstEngParasiticLossesPercentTorque
  Bus Selector9 : BusSelector  OutputSignals=CAN.EC1_00.SPN544_EngineReferenceTorque
  Compare To Zero : simulink/Logic and Bit Operations/Compare To Zero  relop===  OutDataTypeStr=boolean
  ConvertPercentTorqueToNm : Subsystem
  ConvertPercentTorqueToNm1 : Subsystem
  Data Type Conversion{,1..5} (6 alike) : DataTypeConversion  OutDataTypeStr=double
  Determine_engine_torque_and_losses : Subsystem
  Determine_vehicle_speed_and_accel_rate : Subsystem
  Discrete-Time Integrator : DiscreteIntegrator  SampleTime=-1  LimitOutput=on  UpperSaturationLimit=2500  LowerSaturationLimit=0  ICPrevOutput=DiscIntNeverNeededParam  ICPrevScaledInput=DiscIntNeverNeededParam
  F_wheel_to_Tq_eng : MATLAB Function  TreatAsAtomicUnit=on
  If_Then_Else : EmE_MBD_Blockset/Signal Routing/If_Then_Else
      settings: SourceProductName=PACCAR EmE MBD Blockset
  If_Then_Else1 : EmE_MBD_Blockset/Signal Routing/If_Then_Else
      settings: SourceProductName=PACCAR EmE MBD Blockset
  If_Then_Else2 : EmE_MBD_Blockset/Signal Routing/If_Then_Else
      settings: SourceProductName=PACCAR EmE MBD Blockset
  Kff : Gain
  Ki : Gain  Gain=0
  Kp : Gain
  Logical Operator : Logic  Operator=NOT  OutDataTypeStr=boolean
  Logical Operator1 : Logic  Operator=OR  OutDataTypeStr=boolean
  N_rar : Constant  Value=3.25
  Product : Product  InputSameDT=on
  R_wheel_m : Constant  Value=0.5
  Saturation : Saturate  UpperLimit=20  LowerLimit=0.5
  SteadyStateTorqueOffset_Nm : Constant  Value=0
  Subtract : Sum  Inputs=+-  InputSameDT=on
  Subtract1 : Sum  Inputs=+-  InputSameDT=on
  Sum : Sum  Inputs=+++
  Terminator : Terminator
  Terminator1 : Terminator
  TorqueCommandOverride : Constant  Value=false  OutDataTypeStr=boolean
  TorqueCommandOverride_Value_Nm : Constant  Value=0
  UseAccelFBController : Constant  Value=true  OutDataTypeStr=boolean
  UseTorqueFBController : Constant  Value=false  OutDataTypeStr=boolean
  eta : Constant  Value=0.98
  sign : Gain  Gain=-1
  EngineTorque_Nm : Outport
  wires:
  sign/1 -> If_Then_Else2/2
  Logical Operator1/1 -> If_Then_Else2/1
  UseAccelFBController/1 -> Logical Operator1/1
  Logical Operator/1 -> If_Then_Else1/1
  AccelTqTargetKp/1 -> Product/1
  Product/1 -> sign/1  "accel_tq_fb"
  Subtract1/1 -> Product/2  "accel_fb_ctrl_err"
  Determine_vehicle_speed_and_accel_rate/1(Accel_rate_ms2) -> Subtract1/2
  Determine_vehicle_speed_and_accel_rate/2(Vehicle_speed_KPH) -> Terminator1/1
  If_Then_Else2/1 -> Add/2  "accel_tq_fb_out"
  Compare To Zero/1 -> Logical Operator1/2
  AccelFBTqDemDisabled_Nm/1 -> If_Then_Else2/3
  ConvertPercentTorqueToNm/1(EngineParasiticLossesTorque_Nm) -> Add/4
  Bus Selector9/1 -> ConvertPercentTorqueToNm/2(Engine_reference_torque_Nm)  "<SPN544_EngineReferenceTorque>"
  Determine_engine_torque_and_losses/2(Parasitic_losses_torque_pct) -> ConvertPercentTorqueToNm/1(Parasitic_losses_torque_pct)  "Parasitic_losses_torque_pct"
  Bus Selector/1 -> Data Type Conversion/1  "<SPN1760_GrossCombinationVehicleWeight>"
  Bus Selector/2 -> Data Type Conversion1/1  "<SPN526_TransActualGearRatio>"
  SteadyStateTorqueOffset_Nm/1 -> Add/5  "SteadyStateTorqueOffset_Nm"
  Bus Selector8/1 -> Determine_engine_torque_and_losses/1(SPN513_ActualEngPercentTorque)  "<ActualEngPercentTorque>"
  Bus Selector8/2 -> Determine_engine_torque_and_losses/2(SPN4154_ActlEngPrcntTrqueHighResolution)  "<ActlEngPrcntTrqueHighResolution>"
  Bus Selector8/3 -> Determine_engine_torque_and_losses/3(SPN514_NominalFrictionPercentTorque)  "<SPN514_NominalFrictionPercentTorque>"
  Bus Selector8/4 -> Determine_engine_torque_and_losses/4(SPN2978_EstEngParasiticLossesPercentTorque)  "<SPN2978_EstEngParasiticLossesPercentTorque>"
  CAN_In/1 -> Bus Selector8/1, Bus Selector9/1, Determine_vehicle_speed_and_accel_rate/1(In), Bus Selector/1, Bus Selector1/1
  Determine_engine_torque_and_losses/1(Engine_gross_torque_pct) -> Terminator/1
  Saturation/1 -> Accel_target_to_Tq_eng/4(N_tx), F_wheel_to_Tq_eng/4(N_tx)
  F_wheel_to_Tq_eng/1(road_load_tq) -> Add/3
  "RoadLoadEstimate_N "/1 -> F_wheel_to_Tq_eng/1(F_w)
  R_wheel_m/1 -> Data Type Conversion3/1  "R_wheel_m"
  N_rar/1 -> Data Type Conversion4/1  "N_rar"
  eta/1 -> Accel_target_to_Tq_eng/5(eta), Data Type Conversion5/1
  AccelTarget_ms^-2/1 -> Data Type Conversion2/1
  Accel_target_to_Tq_eng/1(accel_tq) -> Compare To Zero/1, Add/1
  Kff/1 -> Sum/1  "FeedForwardTerm"
  Ki/1 -> Sum/3  "IntegralTerm"
  Kp/1 -> Sum/2  "PropTerm"
  Discrete-Time Integrator/1 -> Ki/1
  Sum/1 -> If_Then_Else1/3
  Subtract/1 -> Kp/1, Discrete-Time Integrator/1  "TorqueError_Nm"
  ConvertPercentTorqueToNm1/1(DriverDemandTorque_Nm) -> Subtract/2
  UseTorqueFBController/1 -> Logical Operator/1
  If_Then_Else1/1 -> If_Then_Else/3  "EngineTorque_Nm"
  Bus Selector1/1 -> ConvertPercentTorqueToNm1/1(Driver_demand_torque_pct)  "<DriversDemandEngPercentTorque>"
  Bus Selector1/2 -> ConvertPercentTorqueToNm1/2(Engine_reference_torque_Nm)  "<SPN544_EngineReferenceTorque>"
  Add/1 -> Kff/1, Subtract/1, If_Then_Else1/2  "EngineTorque_Nm"
  TorqueCommandOverride_Value_Nm/1 -> If_Then_Else/2
  TorqueCommandOverride/1 -> If_Then_Else/1
  If_Then_Else/1 -> EngineTorque_Nm/1  "EngineTorque_Nm"
  Data Type Conversion/1 -> Accel_target_to_Tq_eng/1(M)
  Data Type Conversion1/1 -> Saturation/1
  Data Type Conversion2/1 -> Accel_target_to_Tq_eng/6(a_target), Subtract1/1
  Data Type Conversion3/1 -> Accel_target_to_Tq_eng/2(R_w), F_wheel_to_Tq_eng/2(R_w)
  Data Type Conversion4/1 -> Accel_target_to_Tq_eng/3(N_rar), F_wheel_to_Tq_eng/3(N_rar)
  Data Type Conversion5/1 -> F_wheel_to_Tq_eng/5(eta)

== system SUB_L4_Task_10ms_SUB_VELOCITYDISTCTRL/VELOCITYDISTCTRL/TorqueControllerMode/AccelTargetToAcceleratorPosition/EngineTorqueToAccelPedalPos ==
  EngineTorque_Nm : Inport
  Espd_rpm : Inport  Port=2
  2D_Lookup_Table : PTC_MBDS_LIB/Extras/Lookup Tables/2D_Lookup_Table  ParameterObjectName=APTC_TRQ_PED_TRQ_DATA_MPV  InterpolationMethod=Linear  PTC_MBDS_BlockVersion=5.41  PTC_BlockType=PTC_MBDS_2D_Lookup_Table
      settings: SourceProductName=PACCAR Technical Center MBDS Library
      settings: AttributesFormatString=|
      | Row Axis: APTC_TRQ_PED_TRQ_POS_STEP_MPV (%)
      | Column Axis: APTC_TRQ_PED_TRQ_ESPD_STEP_MPV (rpm)
      | Data Axis: APTC_TRQ_PED_TRQ_DATA_MPV (N*m)
      | Interpolation Method: Linear
  Bus Selector : BusSelector  OutputSignals=CAN.EEC1_00.EngSpeed
  Data Type Conversion : DataTypeConversion  OutDataTypeStr=double
      settings: AttributesFormatString=%<OutDataTypeStr>
  AcceleratorPedalPosOut : Outport
  wires:
  Bus Selector/1 -> Data Type Conversion/1  "<EngSpeed>"
  Data Type Conversion/1 -> 2D_Lookup_Table/2
  2D_Lookup_Table/1 -> AcceleratorPedalPosOut/1  "AcceleratorPedalPosOut"
  EngineTorque_Nm/1 -> 2D_Lookup_Table/1
  Espd_rpm/1 -> Bus Selector/1

== system SUB_L4_Task_10ms_SUB_VELOCITYDISTCTRL/VELOCITYDISTCTRL/TorqueControllerMode/AccelTargetToAcceleratorPosition/AccelTargetToEngineTorque/ConvertPercentTorqueToNm ==
  Parasitic_losses_torque_pct : Inport
  Engine_reference_torque_Nm : Inport  Port=2
  Constant2 : Constant  Value=0.01
  Data Type Conversion : DataTypeConversion  OutDataTypeStr=double
  Data Type Conversion1 : DataTypeConversion  OutDataTypeStr=double
  Product : Product  Inputs=3  InputSameDT=on
  EngineParasiticLossesTorque_Nm : Outport
  wires:
  Product/1 -> EngineParasiticLossesTorque_Nm/1  "EngineParasiticLossesTorque_Nm"
  Parasitic_losses_torque_pct/1 -> Data Type Conversion1/1
  Constant2/1 -> Product/1
  Engine_reference_torque_Nm/1 -> Data Type Conversion/1
  Data Type Conversion/1 -> Product/3
  Data Type Conversion1/1 -> Product/2

== system SUB_L4_Task_10ms_SUB_VELOCITYDISTCTRL/VELOCITYDISTCTRL/TorqueControllerMode/AccelTargetToAcceleratorPosition/AccelTargetToEngineTorque/ConvertPercentTorqueToNm1 ==
  Driver_demand_torque_pct : Inport
  Engine_reference_torque_Nm : Inport  Port=2
  Constant2 : Constant  Value=0.01
  Data Type Conversion : DataTypeConversion  OutDataTypeStr=double
      settings: AttributesFormatString=%<OutDataTypeStr>
  Data Type Conversion1 : DataTypeConversion  OutDataTypeStr=double
  Product : Product  Inputs=3  OutDataTypeStr=double  InputSameDT=on
  DriverDemandTorque_Nm : Outport
  wires:
  Data Type Conversion/1 -> Product/2
  Engine_reference_torque_Nm/1 -> Data Type Conversion1/1
  Constant2/1 -> Product/1
  Driver_demand_torque_pct/1 -> Data Type Conversion/1
  Product/1 -> DriverDemandTorque_Nm/1  "DriverDemandTorque_Nm"
  Data Type Conversion1/1 -> Product/3

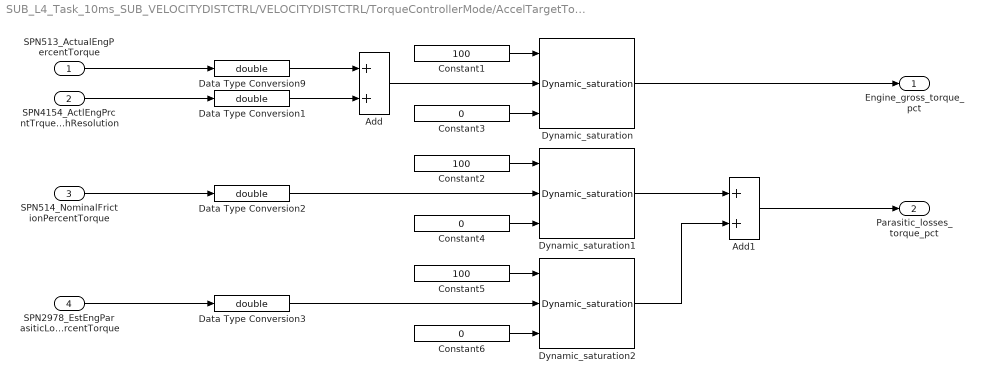
== system SUB_L4_Task_10ms_SUB_VELOCITYDISTCTRL/VELOCITYDISTCTRL/TorqueControllerMode/AccelTargetToAcceleratorPosition/AccelTargetToEngineTorque/Determine_engine_torque_and_losses ==
  SPN513_ActualEngPercentTorque : Inport
  SPN4154_ActlEngPrcntTrqueHighResolution : Inport  Port=2
  SPN514_NominalFrictionPercentTorque : Inport  Port=3
  SPN2978_EstEngParasiticLossesPercentTorque : Inport  Port=4
  Add : Sum  InputSameDT=on
  Add1 : Sum  InputSameDT=on
  Constant1 : Constant  Value=100
  Constant2 : Constant  Value=100
  Constant3 : Constant  Value=0
  Constant4 : Constant  Value=0
  Constant5 : Constant  Value=100
  Constant6 : Constant  Value=0
  Data Type Conversion{1..3,9} (4 alike) : DataTypeConversion  OutDataTypeStr=double  SaturateOnIntegerOverflow=on
  Dynamic_saturation : EmE_MBD_Blockset/Discontinuities/Dynamic_saturation
      settings: SourceProductName=PACCAR EmE MBD Blockset
  Dynamic_saturation1 : EmE_MBD_Blockset/Discontinuities/Dynamic_saturation
      settings: SourceProductName=PACCAR EmE MBD Blockset
  Dynamic_saturation2 : EmE_MBD_Blockset/Discontinuities/Dynamic_saturation
      settings: SourceProductName=PACCAR EmE MBD Blockset
  Engine_gross_torque_pct : Outport
  Parasitic_losses_torque_pct : Outport  Port=2
  wires:
  Data Type Conversion3/1 -> Dynamic_saturation2/2
  Data Type Conversion2/1 -> Dynamic_saturation1/2
  Data Type Conversion1/1 -> Add/2
  Data Type Conversion9/1 -> Add/1
  Add1/1 -> Parasitic_losses_torque_pct/1
  Dynamic_saturation/1 -> Engine_gross_torque_pct/1
  Dynamic_saturation2/1 -> Add1/2
  Dynamic_saturation1/1 -> Add1/1
  Constant5/1 -> Dynamic_saturation2/1
  Constant6/1 -> Dynamic_saturation2/3
  SPN2978_EstEngParasiticLossesPercentTorque/1 -> Data Type Conversion3/1
  Constant2/1 -> Dynamic_saturation1/1
  Constant4/1 -> Dynamic_saturation1/3
  SPN514_NominalFrictionPercentTorque/1 -> Data Type Conversion2/1
  Constant1/1 -> Dynamic_saturation/1
  Constant3/1 -> Dynamic_saturation/3
  Add/1 -> Dynamic_saturation/2
  SPN4154_ActlEngPrcntTrqueHighResolution/1 -> Data Type Conversion1/1
  SPN513_ActualEngPercentTorque/1 -> Data Type Conversion9/1

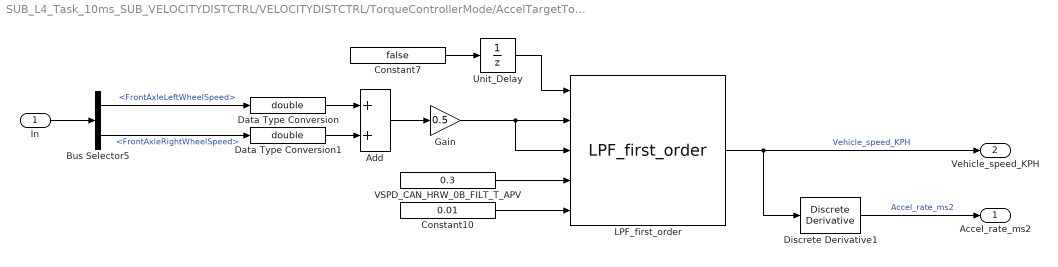
== system SUB_L4_Task_10ms_SUB_VELOCITYDISTCTRL/VELOCITYDISTCTRL/TorqueControllerMode/AccelTargetToAcceleratorPosition/AccelTargetToEngineTorque/Determine_vehicle_speed_and_accel_rate ==
  In : Inport
  Add : Sum  InputSameDT=on
  Bus Selector5 : BusSelector  OutputSignals=CAN.HRW_0B.FrontAxleLeftWheelSpeed,CAN.HRW_0B.FrontAxleRightWheelSpeed
  Constant10 : Constant  Value=0.01
  Constant7 : Constant  Value=false
  Data Type Conversion : DataTypeConversion  OutDataTypeStr=double  SaturateOnIntegerOverflow=on
  Data Type Conversion1 : DataTypeConversion  OutDataTypeStr=double  SaturateOnIntegerOverflow=on
  Discrete Derivative1 : simulink/Discrete/Discrete Derivative  gainval=1.0  ICPrevScaledInput=0.0  InputProcessing=Inherited  OutMin=[]  OutMax=[]  OutDataTypeStr=double  OutputDataTypeScalingMode=double  OutDataType=fixdt(1, 16)  OutScaling=2^-10  DoSatur=off
  Gain : Gain  Gain=0.5  OutDataTypeStr=Inherit: Inherit via back propagation
  LPF_first_order : EmE_MBD_Blockset/Discrete/LPF_first_order
      settings: SourceProductName=PACCAR EmE MBD Blockset
  Unit_Delay : UnitDelay  InitialCondition=true  SampleTime=-1
      settings: AttributesFormatString=IC: %<vinit>
  VSPD_CAN_HRW_0B_FILT_T_APV : Constant  Value=0.3
  Accel_rate_ms2 : Outport
  Vehicle_speed_KPH : Outport  Port=2
  wires:
  VSPD_CAN_HRW_0B_FILT_T_APV/1 -> LPF_first_order/4
  Discrete Derivative1/1 -> Accel_rate_ms2/1  "Accel_rate_ms2"
  Constant10/1 -> LPF_first_order/5
  Add/1 -> Gain/1
  Bus Selector5/2 -> Data Type Conversion1/1  "<FrontAxleRightWheelSpeed>"
  Bus Selector5/1 -> Data Type Conversion/1  "<FrontAxleLeftWheelSpeed>"
  Gain/1 -> LPF_first_order/2, LPF_first_order/3
  Constant7/1 -> Unit_Delay/1
  Unit_Delay/1 -> LPF_first_order/1
  LPF_first_order/1 -> Vehicle_speed_KPH/1, Discrete Derivative1/1  "Vehicle_speed_KPH"
  In/1 -> Bus Selector5/1
  Data Type Conversion/1 -> Add/1
  Data Type Conversion1/1 -> Add/2

== matlab function SUB_L4_Task_10ms_SUB_VELOCITYDISTCTRL/VELOCITYDISTCTRL/TorqueControllerMode/AccelTargetToAcceleratorPosition/AccelTargetToEngineTorque/Accel_target_to_Tq_eng ==
  data: M input; accel_tq output; R_w input; N_rar input; N_tx input; eta input; a_target input
function accel_tq = Accel_target_to_Tq_eng(M, R_w, N_rar, N_tx, eta, a_target)
%#codegen    
    accel_tq = a_target * M * R_w * 1/N_rar * 1/N_tx  * 1/eta;

== matlab function SUB_L4_Task_10ms_SUB_VELOCITYDISTCTRL/VELOCITYDISTCTRL/TorqueControllerMode/AccelTargetToAcceleratorPosition/AccelTargetToEngineTorque/F_wheel_to_Tq_eng ==
  data: F_w input; road_load_tq output; R_w input; N_rar input; N_tx input; eta input
function road_load_tq = F_wheel_to_Tq_eng(F_w, R_w, N_rar, N_tx, eta)
%#codegen    
    road_load_tq = F_w * R_w * 1/N_rar * 1/N_tx * 1/eta;
